simulink model "UAS_Simulink"  (R2021a)
settings: Solver=VariableStepAuto  StartTime=0.0  StopTime=inf  RelTol=1e-3
undefined symbols (not defined in the file or in its folder): Altitude, Latitude, Longitude, Status
libraries: robotlib x5
settings Model: Creator=max  LastModifiedBy=max

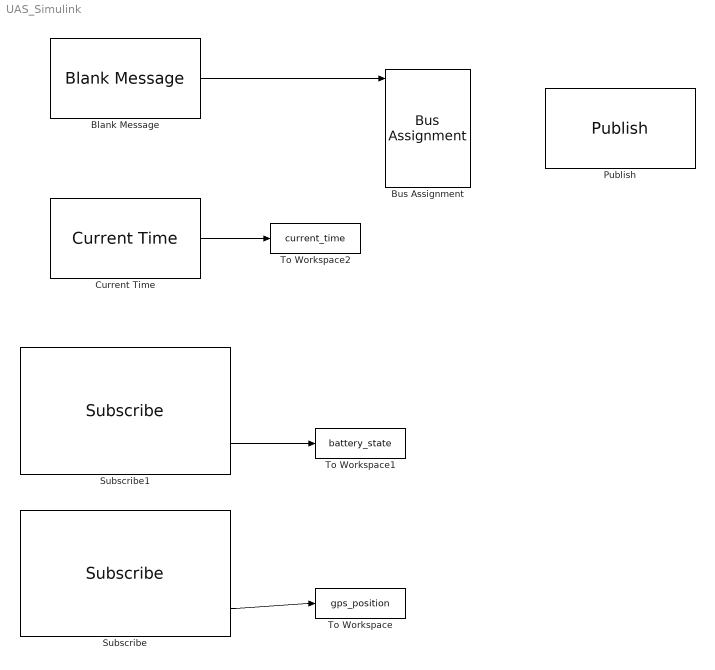
== system UAS_Simulink ==
  Blank Message : robotlib/Blank Message  messageClass=Message  entityType=sensor_msgs/NavSatFix  messageType=sensor_msgs/NavSatFix  SampleTime=inf  legacyBusStruct=off
  Bus Assignment : BusAssignment  AssignedSignals=Latitude,Longitude,Altitude,Status.Status
  Current Time : robotlib/Current Time  OutputFormat=double  SampleTime=-1  ModelName=UAS_Simulink
      settings: SourceProductBaseCode=RR
  Publish : robotlib/Publish  topicSource=Specify your own  topic=/dji_sdk/battery_state  messageType=sensor_msgs/NavSatFix  legacyBusStruct=off  messageQueueLength=1
  Subscribe : robotlib/Subscribe  topicSource=Specify your own  topic=/dji_sdk/gps_position  messageType=sensor_msgs/NavSatFix  SampleTime=-1  legacyBusStruct=off  messageQueueLength=1
  Subscribe1 : robotlib/Subscribe  topicSource=Specify your own  topic=/dji_sdk/battery_state  messageType=sensor_msgs/BatteryState  SampleTime=-1  legacyBusStruct=off  messageQueueLength=1
  To Workspace : ToWorkspace  VariableName=gps_position  SaveFormat=Structure With Time  SampleTime=-1
  To Workspace1 : ToWorkspace  VariableName=battery_state  SampleTime=-1
  To Workspace2 : ToWorkspace  VariableName=current_time  SampleTime=-1
  wires:
  Subscribe/2 -> To Workspace/1
  Subscribe1/2 -> To Workspace1/1
  Current Time/1 -> To Workspace2/1
  Blank Message/1 -> Bus Assignment/1
